simulink model "state_machine"  (R2021a)
settings: Solver=FixedStepAuto  StartTime=0.0  StopTime=10.0  RelTol=1e-3
libraries: slrealtimeutilitieslib x1, slrealtimeiplib x1
settings Model: Creator=Ruixuan  LastModifiedBy=Ruixuan
settings SolverCC: ConcurrentTasks=on  PositivePriorityOrder=on  AutoInsertRateTranBlk=on  InsertRTBMode=Never (minimum delay)
settings OptimizationCC: BlockReduction=off  DefaultParameterBehavior=Inlined  OptimizeBlockIOStorage=off
settings DebuggingCC: TasksWithSamePriorityMsg=none
settings HardwareCC: ProdBitPerLong=64  ProdLongLongMode=on  ProdHWDeviceType=Intel->x86-64 (Linux 64)
settings ModelReferenceCC: ModelReferenceNumInstancesAllowed=Single
settings RTWCC: Description=Simulink Real-Time  SystemTargetFile=slrealtime.tlc  TemplateMakefile=slrealtime_default_tmf  Toolchain=Simulink Real-Time Toolchain  BuildConfiguration=Faster Runs  CodeExecutionProfiling=on  TargetLang=C++

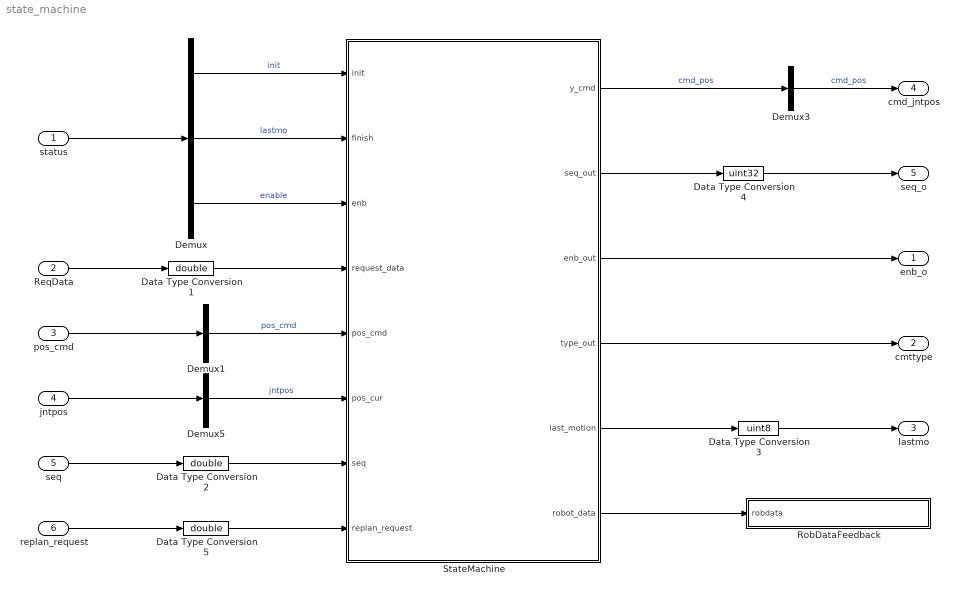
== system state_machine ==
  status : Inport
  ReqData : Inport  Port=2
  pos_cmd : Inport  Port=3
  jntpos : Inport  Port=4
  seq : Inport  Port=5
  replan_request : Inport  Port=6
  Data Type Conversion1 : DataTypeConversion  OutDataTypeStr=double
  Data Type Conversion2 : DataTypeConversion  OutDataTypeStr=double
  Data Type Conversion3 : DataTypeConversion  OutDataTypeStr=uint8
  Data Type Conversion4 : DataTypeConversion  OutDataTypeStr=uint32
  Data Type Conversion5 : DataTypeConversion  OutDataTypeStr=double
  Demux : Demux  Outputs=3
  Demux1 : Demux  Outputs=[21]
  Demux3 : Demux  Outputs=[6]
  Demux5 : Demux  Outputs=[6]
  RobDataFeedback : Subsystem
  StateMachine : MATLAB Function  TreatAsAtomicUnit=on
  enb_o : Outport  VectorParamsAs1DForOutWhenUnconnected=off
  cmttype : Outport  Port=2  VectorParamsAs1DForOutWhenUnconnected=off
  lastmo : Outport  Port=3  VectorParamsAs1DForOutWhenUnconnected=off
  cmd_jntpos : Outport  Port=4  VectorParamsAs1DForOutWhenUnconnected=off
  seq_o : Outport  Port=5  VectorParamsAs1DForOutWhenUnconnected=off
  wires:
  StateMachine/4(type_out) -> cmttype/1
  StateMachine/3(enb_out) -> enb_o/1
  Data Type Conversion4/1 -> seq_o/1
  seq/1 -> Data Type Conversion2/1
  Data Type Conversion3/1 -> lastmo/1
  Demux/2 -> StateMachine/2(finish)  "lastmo"
  StateMachine/1(y_cmd) -> Demux3/1  "cmd_pos"
  jntpos/1 -> Demux5/1
  ReqData/1 -> Data Type Conversion1/1
  status/1 -> Demux/1
  pos_cmd/1 -> Demux1/1
  Demux/3 -> StateMachine/3(enb)  "enable"
  StateMachine/6(robot_data) -> RobDataFeedback/1(robdata)
  Demux/1 -> StateMachine/1(init)  "init"
  Demux1/1 -> StateMachine/5(pos_cmd)  "pos_cmd"
  Demux3/1 -> cmd_jntpos/1  "cmd_pos"
  Data Type Conversion1/1 -> StateMachine/4(request_data)
  Demux5/1 -> StateMachine/6(pos_cur)  "jntpos"
  Data Type Conversion2/1 -> StateMachine/7(seq)
  StateMachine/5(last_motion) -> Data Type Conversion3/1
  StateMachine/2(seq_out) -> Data Type Conversion4/1
  replan_request/1 -> Data Type Conversion5/1
  Data Type Conversion5/1 -> StateMachine/8(replan_request)

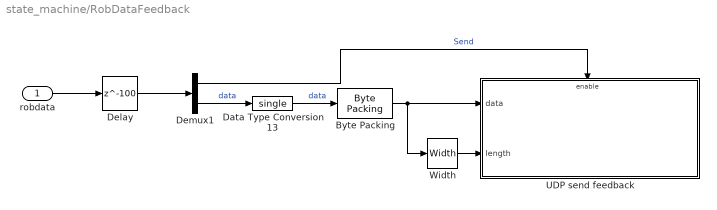
== system state_machine/RobDataFeedback ==
  robdata : Inport
  "Byte Packing " : slrealtimeutilitieslib/Byte Packing  MaskPackedDataType=uint8  MaskUnpackedDataTypes={['single']}  MaskAlignment=1
  Data Type Conversion13 : DataTypeConversion  OutDataTypeStr=single
  Delay : Delay  DelayLength=100  InitialCondition=0
  Demux1 : Demux  Outputs=[1,14]
  UDP send feedback : Subsystem  Priority=100  mask(Stream_send){}
  Width : Width
  wires:
  robdata/1 -> Delay/1
  "Byte Packing "/1 -> Width/1, UDP send feedback/1(data)
  Width/1 -> UDP send feedback/2(length)
  Demux1/2 -> Data Type Conversion13/1  "data"
  Demux1/1 -> UDP send feedback/Enable  "Send"
  Delay/1 -> Demux1/1
  Data Type Conversion13/1 -> "Byte Packing "/1  "data"

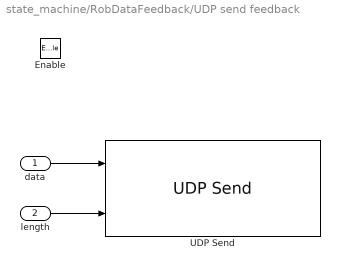
== system state_machine/RobDataFeedback/UDP send feedback ==
  data : Inport
  length : Inport  Port=2
  Enable : EnablePort
  UDP Send : slrealtimeiplib/UDP Send  useHostTargetConn=on  ipAddress=10.10.10.15  localPort=-1  toAddress=192.168.7.2  toPort=25001  sampleTime=Ts
      settings: SourceProductBaseCode=XP
  wires:
  data/1 -> UDP Send/1
  length/1 -> UDP Send/2

== matlab function state_machine/StateMachine ==
  data: init input; finish input; enb input; request_data input; pos_cmd input; pos_cur input; seq input; y_cmd output; seq_out output; enb_out output; type_out output; last_motion output; robot_data output; replan_request input
% This function implements the controller state machine.
% Copyright (C) 2022  
% 
% Authors:
% Ruixuan Liu: ruixuanl@andrew.cmu.edu
% Rui Chen: ruic3@andrew.cmu.edu
% Changliu Liu : cliu6@andrew.cmu.edu
% 
% This program is free software; you can redistribute it and/or
% modify it under the terms of the GNU General Public License
% as published by the Free Software Foundation; either version 2
% of the License, or (at your option) any later version.
% 
% This program is distributed in the hope that it will be useful,
% but WITHOUT ANY WARRANTY; without even the implied warranty of
% MERCHANTABILITY or FITNESS FOR A PARTICULAR PURPOSE.  See the
% GNU General Public License for more details.
% 
% You should have received a copy of the GNU General Public License
% along with this program; if not, write to the Free Software
% Foundation, Inc., 51 Franklin Street, Fifth Floor, Boston, MA  02110-1301, USA.

function [y_cmd, seq_out, enb_out, type_out,...
          last_motion, robot_data] = StateMachine(init, finish, enb, request_data, pos_cmd, pos_cur, seq, replan_request)


    persistent y_pre vel_pre acc_pre seq_pre send_lastmo send_stop;
    persistent m_state;
    
    % Very first recieve. Initialize persistent variables
    if isempty(y_pre)
        [y_pre, vel_pre, acc_pre, seq_pre, send_lastmo, send_stop, m_state] = resetstate(pos_cur);
    end
    task_status = 0;
    
    %% controller logic
    switch enb
        case false
            y_cmd = y_pre;
            seq_out = seq_pre;
            enb_out = 0;
            type_out = 1;
            last_motion = 0;
            if send_lastmo % if need to send last motion
                [type_out, last_motion, enb_out, seq_out, seq_pre, send_stop, send_lastmo] = send_lastmo_cmd(seq, seq_pre);
            elseif send_stop
                % send stop and perform reset
                [type_out, last_motion, enb_out, seq_out] = send_stop_cmd(seq, seq_pre);
                if enb_out % sent stop to robot
                    [~, vel_pre, acc_pre, seq_pre, send_lastmo, send_stop, m_state] = resetstate(pos_cur);
                end
            end
        otherwise
            if init % first packet
                % reset
                [y_pre, vel_pre, acc_pre, seq_pre, send_lastmo, send_stop, m_state] = resetstate(pos_cur);
                [y_cmd, seq_out, enb_out, type_out, last_motion] = send_init_cmd(y_pre, seq_pre, seq);
            elseif finish % if send last motion packet
                [y_cmd, seq_out, seq_pre, enb_out, type_out, last_motion, send_lastmo, send_stop] = send_finish_cmd(y_pre, seq_pre, seq);
            else % if send motion packet
                pos_in = pos_cmd(1:6);
                vel_in = pos_cmd(7:12);
                acc_in = pos_cmd(13:18);
                pos_idx = pos_cmd(19);
                traj_horizon = pos_cmd(20);
                flg = pos_cmd(end);
                if 1 %flg
                    m_state = "posC";
                else
                    m_state = "idle";
                end
                switch m_state
                    case "posC"
                        y_cmd = pos_in(:);
                        y_pre = pos_in(:);
                        vel_pre = vel_in(:);
                        acc_pre = acc_in(:);
                        seq_out = seq_pre;
                        enb_out = 0;
                        type_out = 1;
                        last_motion = 0;
                        task_status = 1;
                        if seq ~= seq_pre % got data
                            seq_out = seq;
                            seq_pre = seq;
                            enb_out = 1;
                        end
                    otherwise % idle
                        y_cmd = y_pre;
                        vel_pre = vel_pre*0;
                        acc_pre = acc_pre*0;
                        seq_out = seq_pre;
                        enb_out = 0;
                        type_out = 1;
                        last_motion = 0;
                        task_status = 0;
                        if seq ~= seq_pre % got data
                            seq_out = seq;
                            seq_pre = seq;
                            enb_out = 1;
                        end
                end
            end
    end

    if request_data % if user request robot status data
        robot_data = [1; pos_cur(:); vel_pre(:); replan_request; task_status];
    else
        robot_data = [0; pos_cur(:); vel_pre(:); replan_request; task_status];
    end
    
    
function [y_cmd, seq_out, seq_pre, enb_out, type_out, last_motion, send_lastmo, send_stop] = send_finish_cmd(y_pre, seq_pre, seq)
    y_cmd = y_pre;
    type_out = 1;
    if seq ~= seq_pre % got data, send
        seq_out = seq;
        seq_pre = seq;
        enb_out = 1;
        last_motion = 1;
        send_lastmo = false;
        send_stop = true;
    else
        seq_out = seq_pre;
        enb_out = 0;
        last_motion = 0;
        send_lastmo = true;
        send_stop = false;
    end
    
    
function [y_cmd, seq_out, enb_out, type_out, last_motion] = send_init_cmd(y_pre, seq_pre, seq)
    y_cmd = y_pre;
    seq_out = seq_pre;
    enb_out = 1;
    type_out = 0;
    last_motion = 0;

    if seq ~= seq_pre
        seq_out = seq;
        seq_pre = seq;
    end
    
    
function [type_out, last_motion, enb_out, seq_out] = send_stop_cmd(seq, seq_pre)
    type_out = 2;
    last_motion = 0;
    enb_out = 0;
    seq_out = seq_pre;
    if seq ~= seq_pre % got data
        enb_out = 1; % send STMO
        seq_out = seq;
    end


function [type_out, last_motion, enb_out, seq_out, seq_pre, send_stop, send_lastmo] = send_lastmo_cmd(seq, seq_pre)
    type_out = 1;
    last_motion = 1;
    enb_out = 0;
    seq_out = seq_pre;
    seq_pre = seq_pre;
    send_stop = true;
    send_lastmo = false;
    if seq ~= seq_pre % got data
        enb_out = 1; % send STMO
        seq_out = seq;
        seq_pre = seq;
    end
    
    
function [y_pre,vel_pre,acc_pre,seq_pre,send_lastmo,send_stop,m_state] = resetstate(pos_cur)
      y_pre = pos_cur(:);
      vel_pre = 0*y_pre(:);
      acc_pre = 0*y_pre(:);
      seq_pre = 0;
      send_lastmo = false;
      send_stop = false;
      m_state = "idle";
